simulink subsystem "Navigation"  (R2023a)
settings: Solver=VariableStepAuto  StartTime=0.0  StopTime=10.0  RelTol=1e-3
settings Model: Creator=Andy  LastModifiedBy=Andy
settings OptimizationCC: ReuseModelBlockBuffer=off
settings ModelReferenceCC: EnableRefExpFcnMdlSchedulingChecks=on

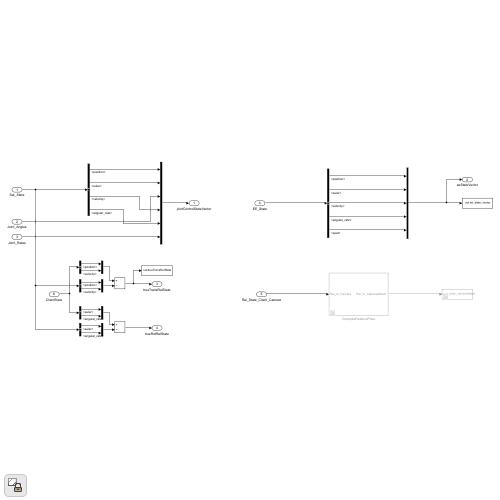
[thumbnail: Simulink's stored preview of the top-level diagram]
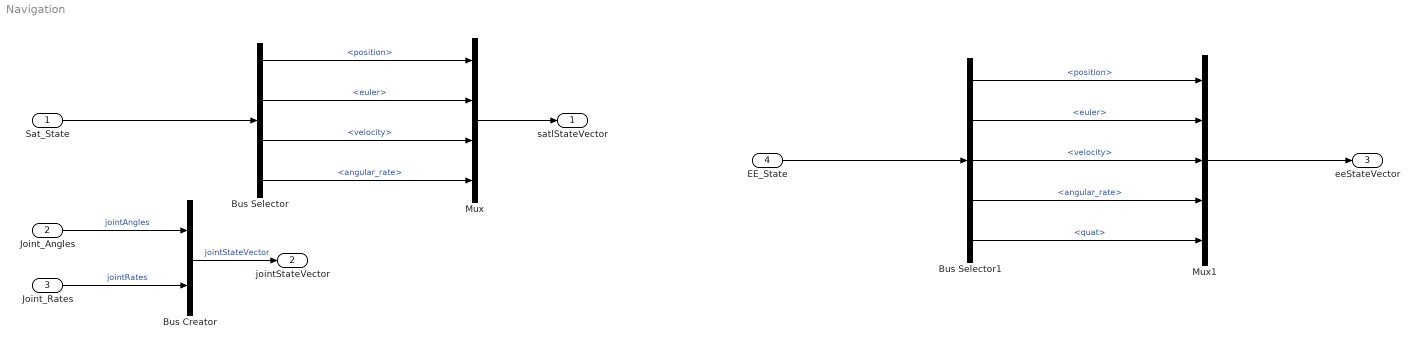
== system Navigation ==
  Sat_State : Inport
  Joint_Angles : Inport  Port=2
  Joint_Rates : Inport  Port=3
  EE_State : Inport  Port=4
  Bus Creator : BusCreator  Inputs=2
  Bus Selector : BusSelector  OutputSignals=translation.position,rotation.euler,translation.velocity,rotation.angular_rate
  Bus Selector1 : BusSelector  OutputSignals=translation.position,rotation.euler,translation.velocity,rotation.angular_rate,rotation.quat
  Mux : Mux
  Mux1 : Mux  Inputs=5
  satlStateVector : Outport
  jointStateVector : Outport  Port=2
  eeStateVector : Outport  Port=3
  wires:
  Mux1/1 -> eeStateVector/1
  Bus Selector/1 -> Mux/1  "<position>"
  Bus Selector/2 -> Mux/2  "<euler>"
  Bus Selector/3 -> Mux/3  "<velocity>"
  Bus Selector/4 -> Mux/4  "<angular_rate>"
  EE_State/1 -> Bus Selector1/1
  Bus Selector1/1 -> Mux1/1  "<position>"
  Bus Selector1/2 -> Mux1/2  "<euler>"
  Sat_State/1 -> Bus Selector/1
  Joint_Rates/1 -> Bus Creator/2  "jointRates"
  Bus Selector1/3 -> Mux1/3  "<velocity>"
  Bus Selector1/4 -> Mux1/4  "<angular_rate>"
  Bus Selector1/5 -> Mux1/5  "<quat>"
  Mux/1 -> satlStateVector/1
  Joint_Angles/1 -> Bus Creator/1  "jointAngles"
  Bus Creator/1 -> jointStateVector/1  "jointStateVector"
